simulink library "NonEntGainCalcBtc"  (R2022b)
settings: Solver=VariableStepAuto  StartTime=0.0  StopTime=10.0  RelTol=1e-3
undefined symbols (not defined in the file or in its folder): Row
libraries: TuneVar x12, TOP x2, FeaturePath x1, HandyTextFile x1, RTC x1, StateVar x1, dspmathops x1
settings Model: Creator=kl13806  LastModifiedBy=kl13806
settings SolverCC: AlgebraicLoopSolver=TrustRegion
settings DebuggingCC: UnconnectedInputMsg=warning  UnconnectedOutputMsg=warning  UnconnectedLineMsg=warning  SFMachineParentedDataDiag=warning
settings ModelReferenceCC: EnableRefExpFcnMdlSchedulingChecks=on
settings RTWCC: DLArmComputeVersion=19.05

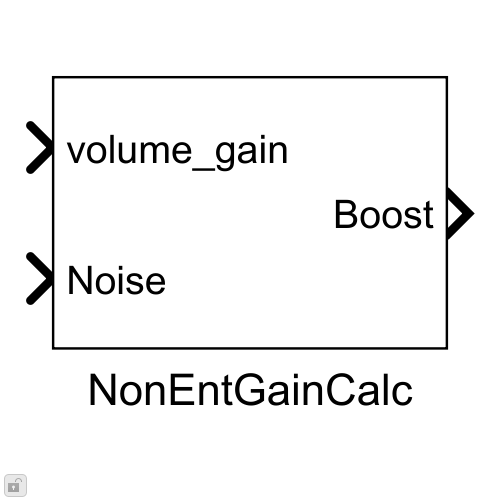
[thumbnail: Simulink's stored preview of the top-level diagram]
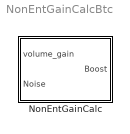
== system NonEntGainCalcBtc ==
  NonEntGainCalc : Subsystem  mask(Blocklib NonEntGainCalc){Config=[], FeatureName=GainCalc}
      mask prompts: Config "NonEntGainCalcConfig"; FeatureName "Feature path name:"
      mask init:
      | blkh=gcbh;
      | Config=BTConfig.Assert(blkh,Config);
      | 
      | Config.Validate();
      | BTConfig.InitSetFeatureIfPresent(blkh,'FeatureName');
      | 
      | % Flatten for MFB is not needed due to mask on MFB. Nice.
      mask Callback Config: BTConfig.CallbackHideIfPresent(gcbh,{'FeatureName'});
      mask TypeOptions FeatureName: FeaturePath/FeatureName
      mask DialogControl ParameterGroupVar2 Prompt: OverRides

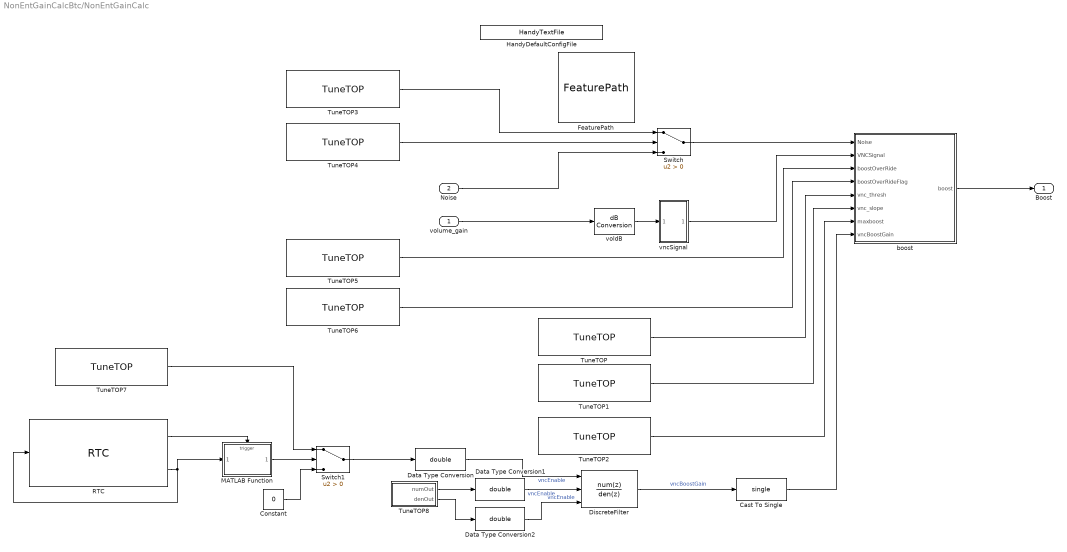
== system NonEntGainCalcBtc/NonEntGainCalc ==
  volume_gain : Inport
  Noise : Inport  Port=2
  Cast To Single : DataTypeConversion  OutDataTypeStr=single  SaturateOnIntegerOverflow=off  RndMeth=Floor
  Constant : Constant  Value=0
  Data Type Conversion : DataTypeConversion  OutDataTypeStr=double  SaturateOnIntegerOverflow=off  RndMeth=Floor
  Data Type Conversion1 : DataTypeConversion  OutDataTypeStr=double  SaturateOnIntegerOverflow=off  RndMeth=Floor
  Data Type Conversion2 : DataTypeConversion  OutDataTypeStr=double  SaturateOnIntegerOverflow=off  RndMeth=Floor
  DiscreteFilter : DiscreteFilter  NumeratorSource=Input port  Numerator=(1-Config.RampCoef)  DenominatorSource=Input port  Denominator=[1 -(Config.RampCoef)]  InputProcessing=Columns as channels (frame based)  FilterStructure=Direct form II transposed  a0EqualsOne=on
      settings: InputPortMap=u0,p1,p3
  FeaturePath : FeaturePath/FeaturePath  FeatureName=GainCalc  IsGroup=off  GroupNumber=-1  IsModule=off  TriggerInit=[-350 -126 -235 -19]
      settings: SourceProductName=Bose Talaria
  HandyDefaultConfigFile : HandyTextFile/HandyTextFile  TemplateSource=Config  FileSuffix=Init  OpenDialogOnLoad=off  UseThisBlockName=off  AddGrandParentNamePrefix=off  TheDefaultText=|  ShowInLibBrowser=on
      | % $(FILENAME) Setup model parameters for each "Init" callback (e.g. update diagram)
      | sample_rate_in_hertz = 44100;
      | frame_size = 32;
      | sysin_channel_count = 2;
      settings: SourceProductName=Bose Talaria
  MATLAB Function : MATLAB Function  TreatAsAtomicUnit=on
  RTC : RTC/RTC  REQ_Priority=RTC_Mask.NormalPriority  RequestAtInit=off  EnableRequest=on  REQElemName1=vncEnable  REQElemType1=uint32  REQElemWidth1=1  REQElemInitial1=0  REQElemType2=uint32  REQElemWidth2=1  REQElemInitial2=[]  REQElemType3=uint32  REQElemWidth3=1  REQElemInitial3=[]  REQElemType4=uint32  REQElemWidth4=1  REQElemInitial4=[]  REQElemType5=uint32  REQElemWidth5=1  REQElemInitial5=[]  REQElemType6=uint32  REQElemWidth6=1  REQElemInitial6=[]  REQElemType7=uint32  REQElemWidth7=1  REQElemInitial7=[]  REQElemType8=uint32  REQElemWidth8=1  REQElemInitial8=[]  REQElemType9=uint32  REQElemWidth9=1  REQElemInitial9=[]  REQElemType10=uint32  REQElemWidth10=1  REQElemInitial10=[]  EnableResponse=on  EnableRSP_StatusIn=off  RSPElemName1=enable  RSPElemType1=uint32  RSPElemWidth1=1  RSPElemType2=uint32  RSPElemWidth2=1  RSPElemType3=uint32  RSPElemWidth3=1  RSPElemType4=uint32  RSPElemWidth4=1  RSPElemType5=uint32  RSPElemWidth5=1  RSPElemType6=uint32  RSPElemWidth6=1  RSPElemType7=uint32  RSPElemWidth7=1  RSPElemType8=uint32  RSPElemWidth8=1  RSPElemType9=uint32  RSPElemWidth9=1  RSPElemType10=uint32  RSPElemWidth10=1  EnableNotification=off  EnableNTF_PrepTrig=off  NTFElemType1=uint32  NTFElemWidth1=1  NTFElemType2=uint32  NTFElemWidth2=1  NTFElemType3=uint32  NTFElemWidth3=1  NTFElemType4=uint32  NTFElemWidth4=1  NTFElemType5=uint32  NTFElemWidth5=1  NTFElemType6=uint32  NTFElemWidth6=1  NTFElemType7=uint32  NTFElemWidth7=1  NTFElemType8=uint32  NTFElemWidth8=1  NTFElemType9=uint32  NTFElemWidth9=1  NTFElemType10=uint32  NTFElemWidth10=1  MaskMessageName=vncEnableRTC
      settings: SourceProductName=Bose Talaria
  Switch : Switch  Criteria=u2 > Threshold  SaturateOnIntegerOverflow=off  InputSameDT=off
  Switch1 : Switch  Criteria=u2 > Threshold  SaturateOnIntegerOverflow=off  InputSameDT=off
  TuneTOP : TuneVar/TuneTOP  TriggerInit=[-380 277 -210 333]  TopName=VncThresh  TuneName=VncThresh  DataType=single  TunabilityNumber=1  MinValue=[]  MaxValue=[]  BankNumber=0  PreOverlay=false  PostOverlay=false  UseSameName=on  MaskValue=Config.DefaultVncThresh
      settings: SourceProductName=Bose Talaria
  TuneTOP1 : TuneVar/TuneTOP  TriggerInit=[-380 347 -210 403]  TopName=VncSlope  TuneName=VncSlope  DataType=single  TunabilityNumber=1  MinValue=[]  MaxValue=[]  BankNumber=0  PreOverlay=false  PostOverlay=false  UseSameName=on  MaskValue=Config.DefaultVncSlope
      settings: SourceProductName=Bose Talaria
  TuneTOP2 : TuneVar/TuneTOP  TriggerInit=[-380 427 -210 483]  TopName=MaxBoost  TuneName=MaxBoost  DataType=single  TunabilityNumber=1  MinValue=[]  MaxValue=[]  BankNumber=0  PreOverlay=false  PostOverlay=false  UseSameName=on  MaskValue=Config.DefaultMaxBoost
      settings: SourceProductName=Bose Talaria
  TuneTOP3 : TuneVar/TuneTOP  TriggerInit=[-760 -98 -590 -42]  TopName=NoiseOverRide  TuneName=NoiseOverRide  DataType=single  TunabilityNumber=1  MinValue=[]  MaxValue=[]  BankNumber=0  PreOverlay=false  PostOverlay=false  UseSameName=on  MaskValue=Config.DefaultNoiseOverride
      settings: SourceProductName=Bose Talaria
  TuneTOP4 : TuneVar/TuneTOP  TriggerInit=[-760 -18 -590 38]  TopName=NoiseOverRideFlag  TuneName=NoiseOverRideFlag  DataType=single  TunabilityNumber=1  MinValue=[]  MaxValue=[]  BankNumber=0  PreOverlay=false  PostOverlay=false  UseSameName=on  MaskValue=Config.DefaultNoiseOverrideFlag
      settings: SourceProductName=Bose Talaria
  TuneTOP5 : TuneVar/TuneTOP  TriggerInit=[-760 157 -590 213]  TopName=BoostOverRide  TuneName=BoostOverRide  DataType=single  TunabilityNumber=1  MinValue=[]  MaxValue=[]  BankNumber=0  PreOverlay=false  PostOverlay=false  UseSameName=on  MaskValue=Config.DefaultBoostOverride
      settings: SourceProductName=Bose Talaria
  TuneTOP6 : TuneVar/TuneTOP  TriggerInit=[-760 232 -590 288]  TopName=BoostOverRideFlag  TuneName=BoostOverRideFlag  DataType=single  TunabilityNumber=1  MinValue=[]  MaxValue=[]  BankNumber=0  PreOverlay=false  PostOverlay=false  UseSameName=on  MaskValue=Config.DefaultBoostOverrideFlag
      settings: SourceProductName=Bose Talaria
  TuneTOP7 : TuneVar/TuneTOP  TriggerInit=[-1110 322 -940 378]  TopName=VncEnableTuneVar  TuneName=VncEnableTuneVar  DataType=single  TunabilityNumber=1  MinValue=[]  MaxValue=[]  BankNumber=0  PreOverlay=false  PostOverlay=false  UseSameName=on  MaskValue=Config.DefaultVncEnable
      settings: SourceProductName=Bose Talaria
  TuneTOP8 : Subsystem
  boost : Subsystem
  vncSignal : Subsystem
  voldB : dspmathops/dB Conversion  dBtype=dB  intype=Amplitude  R=1  fuzz=on
  Boost : Outport  VectorParamsAs1DForOutWhenUnconnected=off
  wires:
  Cast To Single/1 -> boost/8(vncBoostGain)
  Switch/1 -> boost/1(Noise)
  boost/1(boost) -> Boost/1
  TuneTOP2/1 -> boost/7(maxboost)
  TuneTOP1/1 -> boost/6(vnc_slope)
  TuneTOP/1 -> boost/5(vnc_thresh)
  TuneTOP6/1 -> boost/4(boostOverRideFlag)
  TuneTOP5/1 -> boost/3(boostOverRide)
  voldB/1 -> vncSignal/1(In1)
  vncSignal/1(Out1) -> boost/2(VNCSignal)
  volume_gain/1 -> voldB/1
  Noise/1 -> Switch/3
  TuneTOP3/1 -> Switch/1
  TuneTOP4/1 -> Switch/2
  TuneTOP8/1(numOut) -> Data Type Conversion1/1
  TuneTOP8/2(denOut) -> Data Type Conversion2/1
  RTC/1 -> MATLAB Function/Trigger
  Data Type Conversion/1 -> DiscreteFilter/1  "vncEnable"
  RTC/2 -> RTC/1, MATLAB Function/1(vncEnableIn)
  DiscreteFilter/1 -> Cast To Single/1  "vncBoostGain"
  Constant/1 -> Switch1/3
  Switch1/1 -> Data Type Conversion/1
  MATLAB Function/1(vncEnableOut) -> Switch1/2
  TuneTOP7/1 -> Switch1/1
  Data Type Conversion2/1 -> DiscreteFilter/3  "vncEnable"
  Data Type Conversion1/1 -> DiscreteFilter/2  "vncEnable"

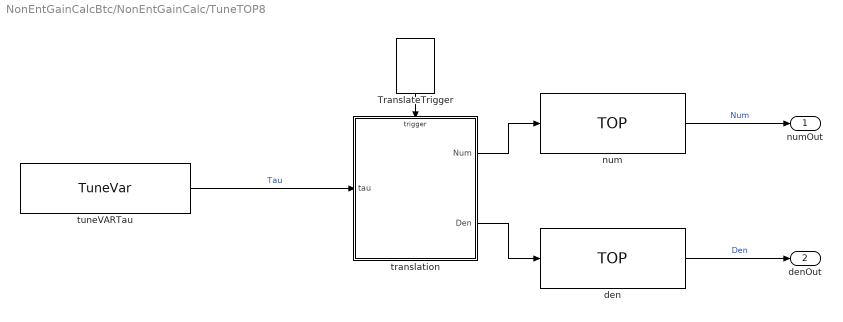
== system NonEntGainCalcBtc/NonEntGainCalc/TuneTOP8 ==
  TranslateTrigger : TuneVar/TranslateTrigger  TriggerInit=[306 -100 344 -45]
      settings: SourceProductName=Bose Talaria
  den : TOP/TOP  TriggerInit=[450 90 595 150]  TopName=Den  DataType=single  BankNumber=0  PreOverlay=false  PostOverlay=false  Role=Automatic
      settings: SourceProductName=Bose Talaria
  num : TOP/TOP  TriggerInit=[450 -45 595 15]  TopName=Num  DataType=single  BankNumber=0  PreOverlay=false  PostOverlay=false  Role=Automatic
      settings: SourceProductName=Bose Talaria
  translation : MATLAB Function  TreatAsAtomicUnit=on  mask{L=Config.FrameSize, Fd=Config.Fd}
  tuneVARTau : TuneVar/TuneVar  TuneName=Tau  SpecifyMaxSize=off  VariableDim=1 (Row)  MaxSize=[1 1]  TunabilityNumber=1  MinValue=[]  MaxValue=[]  TriggerInit=[-70 25 100 75]  MaskValue=Config.DefaultTau
      settings: SourceProductName=Bose Talaria
  numOut : Outport  VectorParamsAs1DForOutWhenUnconnected=off
  denOut : Outport  Port=2  VectorParamsAs1DForOutWhenUnconnected=off
  wires:
  num/1 -> numOut/1  "Num"
  translation/1(Num) -> num/1
  translation/2(Den) -> den/1
  den/1 -> denOut/1  "Den"
  TranslateTrigger/1 -> translation/Trigger
  tuneVARTau/1 -> translation/1(tau)  "Tau"

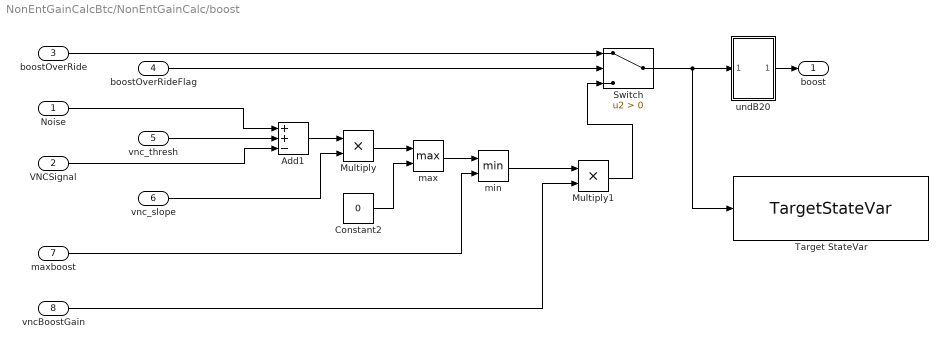
== system NonEntGainCalcBtc/NonEntGainCalc/boost ==
  Noise : Inport
  VNCSignal : Inport  Port=2
  boostOverRide : Inport  Port=3
  boostOverRideFlag : Inport  Port=4
  vnc_thresh : Inport  Port=5
  vnc_slope : Inport  Port=6
  maxboost : Inport  Port=7
  vncBoostGain : Inport  Port=8
  Add1 : Sum  Inputs=++-
  Constant2 : Constant  Value=0  OutDataTypeStr=single
  Multiply : Product
  Multiply1 : Product
  Switch : Switch  Criteria=u2 > Threshold  SaturateOnIntegerOverflow=off  InputSameDT=off
  Target StateVar : StateVar/TargetStateVar  TriggerInit=[655 408 850 472]  TspName=GetNonEntBoostLeveldB  StateName=GetNonEntBoostLeveldB  UseSameName=on  IfdefMacro=[]
      settings: SourceProductName=Bose Talaria
  max : MinMax  Function=max  Inputs=2
  min : MinMax  Inputs=2
  undB20 : Subsystem
  boost : Outport  VectorParamsAs1DForOutWhenUnconnected=off
  wires:
  undB20/1(Out1) -> boost/1
  vnc_slope/1 -> Multiply/2
  vncBoostGain/1 -> Multiply1/2
  maxboost/1 -> min/2
  boostOverRideFlag/1 -> Switch/2
  Multiply/1 -> max/1
  vnc_thresh/1 -> Add1/2
  Constant2/1 -> max/2
  Switch/1 -> Target StateVar/1, undB20/1(In1)
  Noise/1 -> Add1/1
  max/1 -> min/1
  VNCSignal/1 -> Add1/3
  min/1 -> Multiply1/1
  Add1/1 -> Multiply/1
  Multiply1/1 -> Switch/3
  boostOverRide/1 -> Switch/1

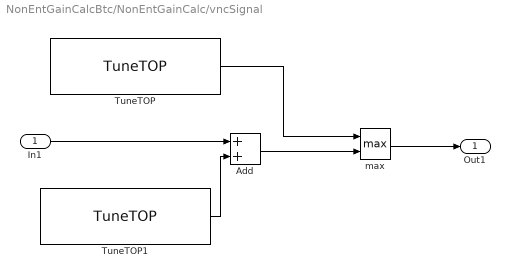
== system NonEntGainCalcBtc/NonEntGainCalc/vncSignal ==
  In1 : Inport
  Add : Sum
  TuneTOP : TuneVar/TuneTOP  TriggerInit=[50 -8 220 48]  TopName=MinVncSignal  TuneName=MinVncSignal  DataType=single  TunabilityNumber=1  MinValue=[]  MaxValue=[]  BankNumber=0  PreOverlay=false  PostOverlay=false  UseSameName=on  MaskValue=Config.DefaultMinVncSignal
      settings: SourceProductName=Bose Talaria
  TuneTOP1 : TuneVar/TuneTOP  TriggerInit=[40 142 210 198]  TopName=MaxSpl  TuneName=MaxSpl  DataType=single  TunabilityNumber=1  MinValue=[]  MaxValue=[]  BankNumber=0  PreOverlay=false  PostOverlay=false  UseSameName=on  MaskValue=Config.DefaultMaxSpl
      settings: SourceProductName=Bose Talaria
  max : MinMax  Function=max  Inputs=2
  Out1 : Outport  VectorParamsAs1DForOutWhenUnconnected=off
  wires:
  max/1 -> Out1/1
  TuneTOP1/1 -> Add/2
  Add/1 -> max/2
  In1/1 -> Add/1
  TuneTOP/1 -> max/1

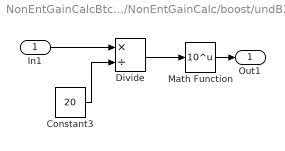
== system NonEntGainCalcBtc/NonEntGainCalc/boost/undB20 ==
  In1 : Inport
  Constant3 : Constant  Value=20  OutDataTypeStr=single
  Divide : Product  Inputs=*/
  Math Function : Math  Operator=10^u  SignedPower=on
  Out1 : Outport  VectorParamsAs1DForOutWhenUnconnected=off
  wires:
  In1/1 -> Divide/1
  Math Function/1 -> Out1/1
  Divide/1 -> Math Function/1
  Constant3/1 -> Divide/2

== matlab function NonEntGainCalcBtc/NonEntGainCalc/MATLAB Function ==
  data: vncEnableIn input; vncEnableOut output
  events: trigger input FUNCTION_CALL_EVENT
function vncEnableOut = fcn(vncEnableIn)
%
%Trivial translation
%
vncEnableOut = vncEnableIn;

== matlab function NonEntGainCalcBtc/NonEntGainCalc/TuneTOP8/translation ==
  data: Num output size=[1,2]; tau input size=1; Den output size=[1,2]; Fd parameter
  events: trigger input FUNCTION_CALL_EVENT
function [Num, Den]  = fcn(tau, Fd)
%
% Calculate coefficients for single pole LPF
%

Wc      = 1/(tau.Value*Fd);
sinCoef = sin(Wc);
cosCoef = cos(Wc);
coef    = (1-sinCoef)/cosCoef;

Num = double([1-coef 0]);
Den =  double([1 -(coef)]);
